simulink library "csc_gdn_guidance_lib"  (R2015b)
settings: Solver=ode45  StartTime=0.0  StopTime=10.0  RelTol=1e-3
undefined symbols (not defined in the file or in its folder): csc_gdn_dt
libraries: util_info_lib x1, csc_cgs_coast_guidance_system_lib x1, csc_gal_gdn_approach_landing_lib x1, csc_gib_gdn_inertial_burn_lib x1, csc_peg_powered_explicit_guidance_lib x1, csu_gml_guidance_mode_logic_lib x1
settings Model: Creator=Nilesh  LastModifiedBy=Mark Agbayani
settings DataIOCC: SaveFormat=Array
settings DebuggingCC: UnderspecifiedInitializationDetection=Classic  MergeDetectMultiDrivingBlocksExec=none  SolverPrmCheckMsg=warning  StateNameClashWarn=warning
settings HardwareCC: ProdBitPerPointer=32  ProdLargestAtomicFloat=None  ProdIntDivRoundTo=Undefined  ProdEndianess=Unspecified  ProdWordSize=32  ProdHWDeviceType=32-bit Generic
settings GRTTargetCC: GeneratePreprocessorConditionals=Disable all
settings ConfigComp: CovModelRefEnable=Off  CovSFcnEnable=off

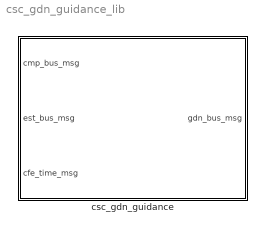
== system csc_gdn_guidance_lib ==
  csc_gdn_guidance : Subsystem  Tag=OFSW; MDL_TICK=EST_BUS_MSG  TreatAsAtomicUnit=on  SystemSampleTime=csc_gdn_dt

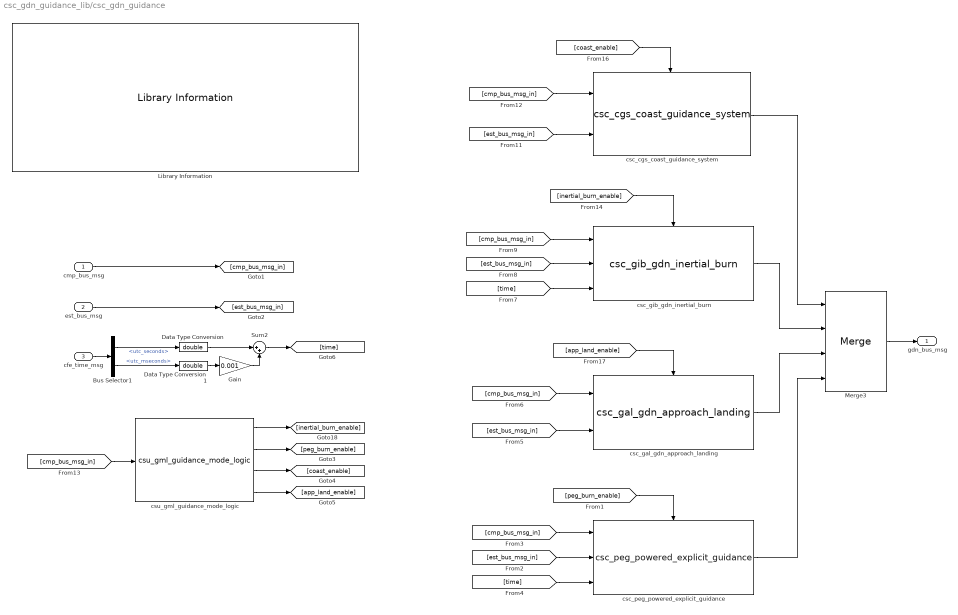
== system csc_gdn_guidance_lib/csc_gdn_guidance ==
  cmp_bus_msg : Inport
  est_bus_msg : Inport  Port=2
  cfe_time_msg : Inport  Port=3  OutDataTypeStr=Bus: cfe_time_msg
  Bus Selector1 : BusSelector  OutputSignals=utc_seconds,utc_mseconds
  Data Type Conversion : DataTypeConversion  OutDataTypeStr=double
  Data Type Conversion1 : DataTypeConversion  OutDataTypeStr=double
  Gain : Gain  Gain=0.001
  Library Information : util_info_lib/Library Information  owner='jkaidy'
  Merge3 : Merge  Inputs=4  InitialOutput=0
  Sum2 : Sum  Inputs=|++
  csc_cgs_coast_guidance_system : csc_cgs_coast_guidance_system_lib/csc_cgs_coast_guidance_system
  csc_gal_gdn_approach_landing : csc_gal_gdn_approach_landing_lib/csc_gal_gdn_approach_landing
  csc_gib_gdn_inertial_burn : csc_gib_gdn_inertial_burn_lib/csc_gib_gdn_inertial_burn
  csc_peg_powered_explicit_guidance : csc_peg_powered_explicit_guidance_lib/csc_peg_powered_explicit_guidance
  csu_gml_guidance_mode_logic : csu_gml_guidance_mode_logic_lib/csu_gml_guidance_mode_logic
  gdn_bus_msg : Outport  OutDataTypeStr=Bus: gdn_bus_msg
  wires:
  [time] -> csc_gib_gdn_inertial_burn/3
  [time] -> csc_peg_powered_explicit_guidance/3
  Sum2/1 -> [time]
  Bus Selector1/2 -> Data Type Conversion1/1  "<utc_mseconds>"
  Data Type Conversion/1 -> Sum2/1
  Data Type Conversion1/1 -> Gain/1
  Gain/1 -> Sum2/2
  Bus Selector1/1 -> Data Type Conversion/1  "<utc_seconds>"
  csc_peg_powered_explicit_guidance/1 -> Merge3/4
  [est_bus_msg_in] -> csc_peg_powered_explicit_guidance/2
  [cmp_bus_msg_in] -> csc_peg_powered_explicit_guidance/1
  [peg_burn_enable] -> csc_peg_powered_explicit_guidance/Enable
  csu_gml_guidance_mode_logic/2 -> [peg_burn_enable]
  cfe_time_msg/1 -> Bus Selector1/1
  csc_gal_gdn_approach_landing/1 -> Merge3/3
  csu_gml_guidance_mode_logic/1 -> [inertial_burn_enable]
  cmp_bus_msg/1 -> [cmp_bus_msg_in]
  est_bus_msg/1 -> [est_bus_msg_in]
  [est_bus_msg_in] -> csc_gal_gdn_approach_landing/2
  [cmp_bus_msg_in] -> csc_gal_gdn_approach_landing/1
  [cmp_bus_msg_in] -> csc_gib_gdn_inertial_burn/1
  [est_bus_msg_in] -> csc_gib_gdn_inertial_burn/2
  [cmp_bus_msg_in] -> csc_cgs_coast_guidance_system/1
  [est_bus_msg_in] -> csc_cgs_coast_guidance_system/2
  csu_gml_guidance_mode_logic/3 -> [coast_enable]
  csu_gml_guidance_mode_logic/4 -> [app_land_enable]
  [cmp_bus_msg_in] -> csu_gml_guidance_mode_logic/1
  [app_land_enable] -> csc_gal_gdn_approach_landing/Enable
  [inertial_burn_enable] -> csc_gib_gdn_inertial_burn/Enable
  [coast_enable] -> csc_cgs_coast_guidance_system/Enable
  csc_gib_gdn_inertial_burn/1 -> Merge3/2
  csc_cgs_coast_guidance_system/1 -> Merge3/1
  Merge3/1 -> gdn_bus_msg/1
